simulink library "xpcdiamondlib"  (Simulink 6.0)
settings: Solver=ode45  SolverMode=SingleTasking  StartTime=0.0  StopTime=10.0  RelTol=1e-3
values from neighbouring files (symbols this model uses):
  channel = Channels(i)    [madadvpcl812.m]    (also in madadvpcl818.m; madhsad512.m; madsbsip16adc.m = round(channel); madsbsiphiadc.m = round(channel))
undefined symbols (not defined in the file or in its folder): maddiamondmm, maddiamondmm32, maddiamondmm32frame, maddsmm16at, madprometheus, mdadiamondmm, mdadiamondmmx, mdadsmm16at, mdaprometheus, mdidiamondmm, mdiodiamondquartz, mdiodsmm, mdodiamondmm, mdsrubymm, mdsrubymm1612, mdsrubymm416, misa8255
libraries: xpcmeasurementcomputinglib x12
(part 2 of 2)

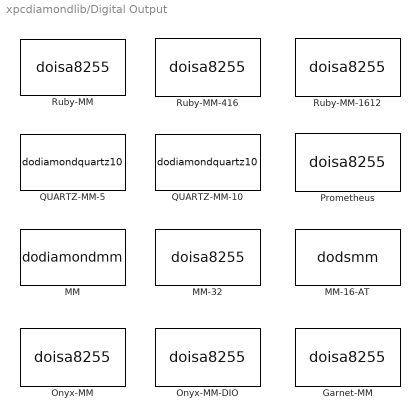
== system xpcdiamondlib/Digital Output ==
  "Garnet-MM " : S-Function  InitFcn=misa8255(1)  FunctionName=doisa8255  Parameters=channel, port, reset, initValue, sampletime, baseaddress, control  mask(dodsgarnetmm){channel=[1], port=A, reset=[1], initValue=[0], chip=1, sampletime=.001, baseaddress=0x300}
      mask prompts: channel "Channel vector:"; reset "Reset vector:"; initValue "Initial value vector:"; sampletime "Sample time:"; baseaddress "Base address (e.g. 0x300):"
      mask help:
      | Garnet-MM
      | Diamond Systems
      | Digital Output
      mask init:
      | baseaddress=hex2dec(baseaddress(3:end));
      | control=155;
      | [baseaddress,control,maskdisplay,maskdescription,reset,initValue]=misa8255(2, chip, port, channel, baseaddress, reset, initValue);
      | set_param(gcb, 'MaskDisplay', maskdisplay);
      | set_param(gcb, 'MaskDescription', maskdescription);
      mask Help: helpview(fullfile(docroot, 'mapfiles', 'xpc.map'), 'Diamond_Garnet-MM_DOUT')
      mask StyleString: edit,popup(A|B|C),edit,edit,popup(1|2),edit,edit
      mask Display: disp('Garnet-MM\nDiamond\nDigital Output');port_label('input',1,'1');
  "MM " : S-Function  InitFcn=mdodiamondmm(1);  FunctionName=dodiamondmm  Parameters=channel, reset, initValue, sampleTime, baseDec  mask(dodiamondmm){channel=[1], reset=[0 ], initValue=[1 ], sampleTime=0.001, base=0x300}
      mask prompts: channel "Channel vector:"; reset "Reset vector:"; initValue "Initial value vector:"; sampleTime "Sample time:"; base "Base address (e.g. 0x300):"
      mask help:
      | MM
      | Diamond
      | Digital Output
      mask init:
      | phase = 2;
      | [reset, initValue, baseDec, maskDisplay, maskDescription] = mdodiamondmm(phase, channel, reset, initValue, sampleTime, base);
      | set_param(gcb, 'MaskDisplay', maskDisplay);
      | set_param(gcb, 'MaskDescription', maskDescription);
      mask Help: helpview(fullfile(docroot, 'mapfiles', 'xpc.map'), 'Diamond_MM_DOUT')
      mask Display: disp('MM\nDiamond\nDigital Output'); port_label('input', 1, '1');
  "MM-16-AT " : S-Function  InitFcn=mdiodsmm(1, 'MM-16-AT', 'output');  FunctionName=dodsmm  Parameters=channel, reset, initValue, sampleTime, baseDec  mask(dodiamondmm16at){channel=[1], reset=[0 ], initValue=[1 ], sampleTime=0.001, baseHex=0x300}
      mask prompts: channel "Channel vector:"; reset "Reset vector:"; initValue "Initial value vector:"; sampleTime "Sample time:"; baseHex "Base address (e.g. 0x300):"
      mask help:
      | MM-16-AT
      | Diamond
      | Digital Output
      mask init:
      | phase = 2;
      | deviceName = 'MM-16-AT';
      | direction = 'output';
      | [baseDec, maskDisplay, maskDescription, reset, initValue] = mdiodsmm(phase, deviceName, direction, channel, sampleTime, baseHex, reset, initValue);
      | set_param(gcb, 'MaskDisplay', maskDisplay);
      | set_param(gcb, 'MaskDescription', maskDescription);
      mask Help: helpview(fullfile(docroot, 'mapfiles', 'xpc.map'), 'Diamond_MM-16-AT_DOUT')
      mask Display: disp('MM-16-AT\nDiamond\nDigital Output'); port_label('input', 1, '1');
  "MM-32 " : S-Function  InitFcn=misa8255(1)  FunctionName=doisa8255  Parameters=channel, port, reset, initValue, sampletime, baseaddress, control  mask(dodsmm32){channel=[1], port=A, reset=[1], initValue=[0], chip=1, sampletime=0.001, baseaddress=0x300}
      mask prompts: channel "Channel vector:"; reset "Reset vector:"; initValue "Initial value vector:"; sampletime "Sample time:"; baseaddress "Base address (i.e. 0xd000):"
      mask help:
      | MM-32
      | Diamond Systems
      | Digital Output
      mask init:
      | baseaddress=hex2dec(baseaddress(3:end));
      | control=155;
      | boardType=16;
      | [baseaddress,control,maskdisplay,maskdescription,reset,initValue]=misa8255(2, chip, port, channel, baseaddress, reset, initValue);
      | set_param(gcb, 'MaskDisplay', maskdisplay);
      | set_param(gcb, 'MaskDescription', maskdescription);
      mask Help: helpview(fullfile(docroot, 'mapfiles', 'xpc.map'), 'Diamond_MM-32_DOUT')
      mask StyleString: edit,popup(A|B|C),edit,edit,popup(1),edit,edit
      mask Display: disp('MM-32\nDiamond\nDigital Output');port_label('input',1,'1');
  "Onyx-MM " : S-Function  InitFcn=misa8255(1)  FunctionName=doisa8255  Parameters=channel, port, reset, initValue, sampletime, baseaddress, control  mask(dodsonyxmm){channel=[1], port=A, reset=[1], initValue=[0], chip=1, sampletime=.001, baseaddress=0x300}
      mask prompts: channel "Channel vector:"; reset "Reset vector:"; initValue "Initial value vector:"; sampletime "Sample time:"; baseaddress "Base address (e.g. 0x300):"
      mask help:
      | Onyx-MM
      | Diamond Systems
      | Digital Output
      mask init: same as xpcdiamondlib/Digital Output/MM-32 
      mask Help: helpview(fullfile(docroot, 'mapfiles', 'xpc.map'), 'Diamond_Onyx-MM_DOUT')
      mask StyleString: edit,popup(A|B|C),edit,edit,popup(1|2),edit,edit
      mask Display: disp('Onyx-MM\nDiamond\nDigital Output');port_label('input',1,'1');
  "Onyx-MM-DIO " : S-Function  InitFcn=misa8255(1)  FunctionName=doisa8255  Parameters=channel, port, reset, initValue, sampletime, baseaddress, control  mask(dodsonyxmmdio){channel=[1], port=A, reset=[1], initValue=[0], chip=1, sampletime=.001, baseaddress=0x300}
      mask prompts: channel "Channel vector:"; reset "Reset vector:"; initValue "Initial value vector:"; sampletime "Sample time:"; baseaddress "Base address (e.g. 0x300):"
      mask help:
      | Onyx-MM-DIO
      | Diamond Systems
      | Digital Output
      mask init: same as xpcdiamondlib/Digital Output/Garnet-MM 
      mask Help: helpview(fullfile(docroot, 'mapfiles', 'xpc.map'), 'Diamond_Onyx-MM-DIO_DOUT')
      mask StyleString: edit,popup(A|B|C),edit,edit,popup(1|2),edit,edit
      mask Display: disp('Onyx-MM-DIO\nDiamond\nDigital Output');port_label('input',1,'1');
  Prometheus : S-Function  InitFcn=misa8255(1)  FunctionName=doisa8255  Parameters=channel, port, reset, initValue, sampletime, baseaddress, control  mask(dodsprometheus){channel=[1], port=B, reset=[1], initValue=[0 ], chip=1, sampletime=0.001, baseaddress=0x280}
      mask prompts: channel "Channel vector:"; reset "Reset vector:"; initValue "Initial value vector:"; sampletime "Sample time:"; baseaddress "Base address (e.g. 0x280):"
      mask help:
      | Prometheus
      | Diamond Systems
      | Digital Output
      mask init: same as xpcdiamondlib/Digital Output/MM-32 
      mask Help: helpview(fullfile(docroot, 'mapfiles', 'xpc.map'), 'Diamond_Prometheus_DOUT')
      mask StyleString: edit,popup(A|B|C),edit,edit,popup(1),edit,edit
      mask Display: disp('Prometheus\nDiamond\nDigital Output');port_label('input',1,'1');
  "QUARTZ-MM-10 " : S-Function  InitFcn=mdiodiamondquartz(1);  FunctionName=dodiamondquartz10  Parameters=channel, ts, baseAddress  mask(dodiamondquartz10){channel=[1], ts=0.001, baseAddressIn=0x300}
      mask prompts: channel "Channel vector:"; ts "Sample time:"; baseAddressIn "Base address (i.e. 0xd000):"
      mask help:
      | QUARTZ-MM-10
      | Diamond Systems
      | Digital Output
      mask init:
      | type=1;
      | baseAddress=768;
      | [baseAddress, maskdisplay,maskdescription]=mdiodiamondquartz(2, type, channel, baseAddressIn);
      | set_param(gcb,'MaskDisplay',maskdisplay);
      | set_param(gcb,'MaskDescription',maskdescription);
      mask Help: helpview(fullfile(docroot, 'mapfiles', 'xpc.map'), 'Diamond_QUARTZ-MM-10_DOUT')
      mask Display: disp('Quartz-MM-10\nDiamond\nDigital Output'); port_label('input', 1, '1');
  "QUARTZ-MM-5 " : S-Function  InitFcn=mdiodiamondquartz(1);  FunctionName=dodiamondquartz10  Parameters=channel, ts, baseAddress  mask(dodiamondquartz10){channel=[1], ts=0.001, baseAddressIn=0x300}
      mask prompts: channel "Channel vector:"; ts "Sample time:"; baseAddressIn "Base address (i.e. 0xd000):"
      mask help:
      | Quartz-MM-5
      | Diamond
      | Digital Output
      mask init:
      | type=3;
      | baseAddress=768;
      | [baseAddress, maskdisplay,maskdescription]=mdiodiamondquartz(2, type, channel, baseAddressIn);
      | set_param(gcb,'MaskDisplay',maskdisplay);
      | set_param(gcb,'MaskDescription',maskdescription);
      mask Help: helpview(fullfile(docroot, 'mapfiles', 'xpc.map'), 'Diamond_QUARTZ-MM-5_DOUT')
      mask Display: disp('Quartz-MM-5\nDiamond\nDigital Output'); port_label('input', 1, '1');
  "Ruby-MM " : S-Function  InitFcn=misa8255(1)  FunctionName=doisa8255  Parameters=channel, port, reset, initValue, sampletime, baseaddress, control  mask(dodsrubymm){channel=[1], port=A, reset=[1], initValue=[0], chip=1, sampletime=0.001, baseaddress=0x300}
      mask prompts: channel "Channel vector:"; reset "Reset vector:"; initValue "Initial value vector:"; sampletime "Sample time:"; baseaddress "Base address (i.e. 0xd000):"
      mask help:
      | Ruby-MM
      | Diamond Systems
      | Digital Output
      mask init: same as xpcdiamondlib/Digital Output/Garnet-MM 
      mask Help: helpview(fullfile(docroot, 'mapfiles', 'xpc.map'), 'Diamond_Ruby-MM_DOUT')
      mask StyleString: edit,popup(A|B|C),edit,edit,popup(1),edit,edit
      mask Display: disp('Ruby-MM\nDiamond\nDigital Output');port_label('input',1,'1');
  "Ruby-MM-1612 " : S-Function  InitFcn=misa8255(1)  FunctionName=doisa8255  Parameters=channel, port, reset, initValue, sampletime, baseaddress, control  mask(dodsrubymm1612){channel=[1], port=A, reset=[1], initValue=[0], chip=1, sampletime=.001, baseaddress=0x300}
      mask prompts: channel "Channel vector:"; reset "Reset vector:"; initValue "Initial value vector:"; sampletime "Sample time:"; baseaddress "Base address (e.g. 0x300):"
      mask help:
      | Ruby-MM-1612
      | Diamond Systems
      | Digital Output
      mask init: same as xpcdiamondlib/Digital Output/MM-32 
      mask Help: helpview(fullfile(docroot, 'mapfiles', 'xpc.map'), 'Diamond_Ruby-MM-1612_DOUT')
      mask StyleString: edit,popup(A|B|C),edit,edit,popup(1),edit,edit
      mask Display: disp('Ruby-MM-1612\nDiamond\nDigital Output');port_label('input',1,'1');
  "Ruby-MM-416 " : S-Function  InitFcn=misa8255(1)  FunctionName=doisa8255  Parameters=channel, port, reset, initValue, sampletime, baseaddress, control  mask(dodsrubymm416){channel=[1], port=A, reset=[1], initValue=[0], chip=1, sampletime=.001, baseaddress=0x300}
      mask prompts: channel "Channel vector:"; reset "Reset vector:"; initValue "Initial value vector:"; sampletime "Sample time:"; baseaddress "Base address (e.g. 0x300):"
      mask help:
      | Ruby-MM-416
      | Diamond Systems
      | Digital Output
      mask init: same as xpcdiamondlib/Digital Output/MM-32 
      mask Help: helpview(fullfile(docroot, 'mapfiles', 'xpc.map'), 'Diamond_Ruby-MM-416_DOUT')
      mask StyleString: edit,popup(A|B|C),edit,edit,popup(1),edit,edit
      mask Display: disp('Ruby-MM-416\nDiamond\nDigital Output');port_label('input',1,'1');

== system xpcdiamondlib/RS232 ==

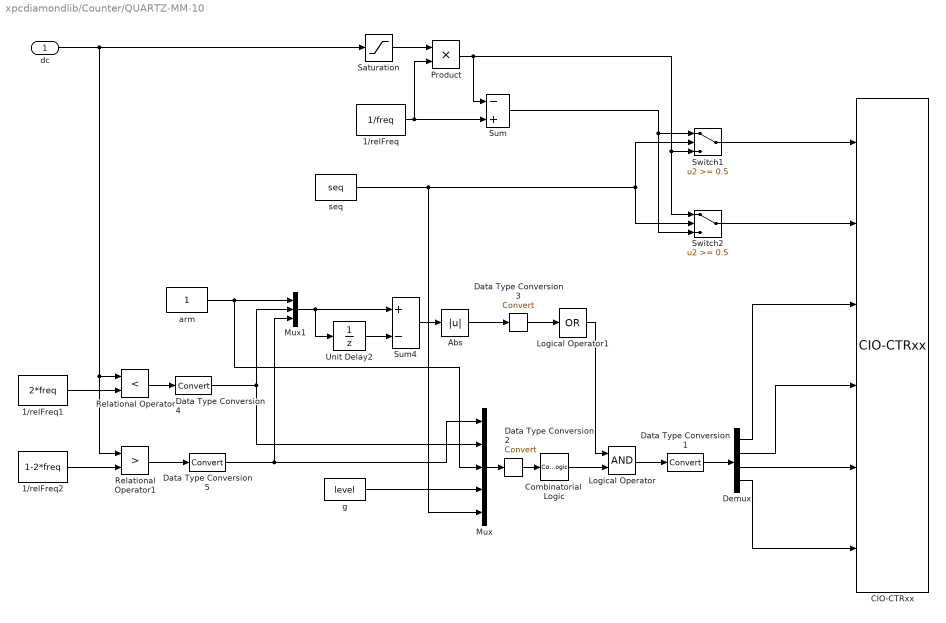
== system xpcdiamondlib/Counter/QUARTZ-MM-10  ==
  dc : Inport  LatchInput=off
  1/relFreq : Constant  Value=1/freq
  1/relFreq1 : Constant  Value=2*freq
  1/relFreq2 : Constant  Value=1-2*freq
  Abs : Abs  SaturateOnIntegerOverflow=on
  "CIO-CTRxx " : xpcmeasurementcomputinglib/Counter/CIO-CTRxx   mastermode=MasterMode  countermode=CounterMode  init=Init  commands=Runtime  term=Term  ts=Ts  baseAddress=baseAddress
  Combinatorial  Logic : CombinatorialLogic  TruthTable=[0,0,1,0;0,0,1,0;0,0,0,1;0,0,0,1;0,1,0,0;1,0,0,0;0,1,0,0;1,0,0,0;0,0,1,0;0,0,1,0;0,0,0,1;0,0,0,1;0,0,1,0;0,0,1,0;0,0,1,0;0,0,1,0;0,0,1,0;0,0,1,0;0,0,0,1;0,0,0,1;0,0,0,1;0,0,0,1;0,0,0,1;0,0,0,1;0,0,0,0;0,0,0,0;0,0,0,0;0,0,0,0;0,0,0,0;0,0,0,0;0,0,0,0;0,0,0,0]
  Data Type Conversion1 : DataTypeConversion  SaturateOnIntegerOverflow=on  RndMeth=Zero
  Data Type Conversion2 : DataTypeConversion  SaturateOnIntegerOverflow=on  RndMeth=Zero
  Data Type Conversion3 : DataTypeConversion  SaturateOnIntegerOverflow=on  RndMeth=Zero
  Data Type Conversion4 : DataTypeConversion  OutDataTypeMode=double  SaturateOnIntegerOverflow=on  RndMeth=Zero
  Data Type Conversion5 : DataTypeConversion  OutDataTypeMode=double  SaturateOnIntegerOverflow=on  RndMeth=Zero
  Demux : Demux
  Logical Operator : Logic
  Logical Operator1 : Logic  Operator=OR  Inputs=1
  Mux : Mux  Inputs=5
  Mux1 : Mux  Inputs=3
  Product : Product  SaturateOnIntegerOverflow=on  InputSameDT=on
  Relational Operator : RelationalOperator  Operator=<  InputSameDT=on
  Relational Operator1 : RelationalOperator  Operator=>  InputSameDT=on
  Saturation : Saturate  UpperLimit=1-2*freq  LowerLimit=2*freq  ZeroCross=off
  Sum : Sum  Inputs=-+  SaturateOnIntegerOverflow=on  InputSameDT=on
  Sum4 : Sum  Inputs=+-  SaturateOnIntegerOverflow=on  InputSameDT=on
  Switch1 : Switch  Threshold=0.5  InputSameDT=on
  Switch2 : Switch  Threshold=0.5  InputSameDT=on
  Unit Delay2 : UnitDelay  X0=2  SampleTime=Ts
  arm : Constant
  g : Constant  Value=level
  seq : Constant  Value=seq
  wires:
  Data Type Conversion5/1 -> Mux1/3, Mux/1
  Data Type Conversion4/1 -> Mux1/2, Mux/2
  Data Type Conversion3/1 -> Logical Operator1/1
  Data Type Conversion2/1 -> Combinatorial  Logic/1
  Data Type Conversion1/1 -> Demux/1
  1/relFreq1/1 -> Relational Operator/2
  1/relFreq/1 -> Product/2, Sum/2
  Product/1 -> Sum/1, Switch1/3, Switch2/1
  1/relFreq2/1 -> Relational Operator1/2
  Relational Operator1/1 -> Data Type Conversion5/1
  Relational Operator/1 -> Data Type Conversion4/1
  Combinatorial  Logic/1 -> Logical Operator/2
  Logical Operator/1 -> Data Type Conversion1/1
  Unit Delay2/1 -> Sum4/2
  Sum4/1 -> Abs/1
  Logical Operator1/1 -> Logical Operator/1
  Demux/1 -> "CIO-CTRxx "/3
  Demux/2 -> "CIO-CTRxx "/4
  Demux/3 -> "CIO-CTRxx "/5
  Demux/4 -> "CIO-CTRxx "/6
  g/1 -> Mux/4
  seq/1 -> Switch1/2, Switch2/2, Mux/5
  Sum/1 -> Switch1/1, Switch2/3
  Saturation/1 -> Product/1
  dc/1 -> Saturation/1, Relational Operator/1, Relational Operator1/1
  Mux1/1 -> Sum4/1, Unit Delay2/1
  arm/1 -> Mux1/1, Mux/3
  Abs/1 -> Data Type Conversion3/1
  Mux/1 -> Data Type Conversion2/1
  Switch1/1 -> "CIO-CTRxx "/1
  Switch2/1 -> "CIO-CTRxx "/2

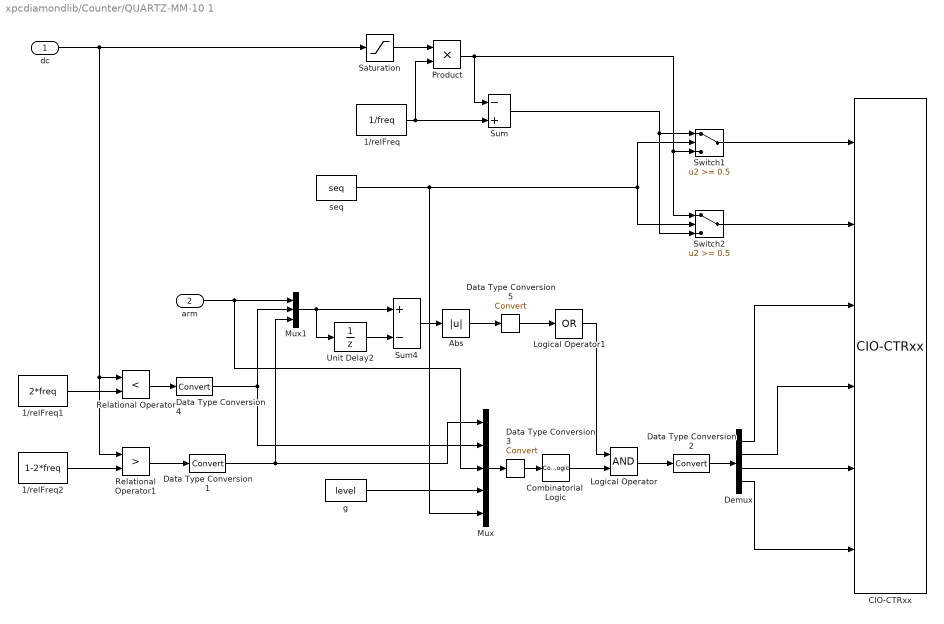
== system xpcdiamondlib/Counter/QUARTZ-MM-10 1 ==
  dc : Inport  LatchInput=off
  arm : Inport  Port=2  LatchInput=off
  1/relFreq : Constant  Value=1/freq
  1/relFreq1 : Constant  Value=2*freq
  1/relFreq2 : Constant  Value=1-2*freq
  Abs : Abs  SaturateOnIntegerOverflow=on
  "CIO-CTRxx " : xpcmeasurementcomputinglib/Counter/CIO-CTRxx   mastermode=MasterMode  countermode=CounterMode  init=Init  commands=Runtime  term=Term  ts=Ts  baseAddress=baseAddress
  Combinatorial  Logic : CombinatorialLogic  TruthTable=[0,0,1,0;0,0,1,0;0,0,0,1;0,0,0,1;0,1,0,0;1,0,0,0;0,1,0,0;1,0,0,0;0,0,1,0;0,0,1,0;0,0,0,1;0,0,0,1;0,0,1,0;0,0,1,0;0,0,1,0;0,0,1,0;0,0,1,0;0,0,1,0;0,0,0,1;0,0,0,1;0,0,0,1;0,0,0,1;0,0,0,1;0,0,0,1;0,0,0,0;0,0,0,0;0,0,0,0;0,0,0,0;0,0,0,0;0,0,0,0;0,0,0,0;0,0,0,0]
  Data Type Conversion1 : DataTypeConversion  OutDataTypeMode=double  SaturateOnIntegerOverflow=on  RndMeth=Zero
  Data Type Conversion2 : DataTypeConversion  SaturateOnIntegerOverflow=on  RndMeth=Zero
  Data Type Conversion3 : DataTypeConversion  SaturateOnIntegerOverflow=on  RndMeth=Zero
  Data Type Conversion4 : DataTypeConversion  OutDataTypeMode=double  SaturateOnIntegerOverflow=on  RndMeth=Zero
  Data Type Conversion5 : DataTypeConversion  SaturateOnIntegerOverflow=on  RndMeth=Zero
  Demux : Demux
  Logical Operator : Logic
  Logical Operator1 : Logic  Operator=OR  Inputs=1
  Mux : Mux  Inputs=5
  Mux1 : Mux  Inputs=3
  Product : Product  SaturateOnIntegerOverflow=on  InputSameDT=on
  Relational Operator : RelationalOperator  Operator=<  InputSameDT=on
  Relational Operator1 : RelationalOperator  Operator=>  InputSameDT=on
  Saturation : Saturate  UpperLimit=1-2*freq  LowerLimit=2*freq  ZeroCross=off
  Sum : Sum  Inputs=-+  SaturateOnIntegerOverflow=on  InputSameDT=on
  Sum4 : Sum  Inputs=+-  SaturateOnIntegerOverflow=on  InputSameDT=on
  Switch1 : Switch  Threshold=0.5  InputSameDT=on
  Switch2 : Switch  Threshold=0.5  InputSameDT=on
  Unit Delay2 : UnitDelay  X0=2  SampleTime=Ts
  g : Constant  Value=level
  seq : Constant  Value=seq
  wires:
  Data Type Conversion5/1 -> Logical Operator1/1
  Data Type Conversion3/1 -> Combinatorial  Logic/1
  Data Type Conversion2/1 -> Demux/1
  Data Type Conversion1/1 -> Mux1/3, Mux/1
  Data Type Conversion4/1 -> Mux1/2, Mux/2
  1/relFreq1/1 -> Relational Operator/2
  1/relFreq/1 -> Product/2, Sum/2
  Product/1 -> Sum/1, Switch1/3, Switch2/1
  1/relFreq2/1 -> Relational Operator1/2
  Relational Operator1/1 -> Data Type Conversion1/1
  Relational Operator/1 -> Data Type Conversion4/1
  Combinatorial  Logic/1 -> Logical Operator/2
  Logical Operator/1 -> Data Type Conversion2/1
  Unit Delay2/1 -> Sum4/2
  Sum4/1 -> Abs/1
  Logical Operator1/1 -> Logical Operator/1
  Demux/1 -> "CIO-CTRxx "/3
  Demux/2 -> "CIO-CTRxx "/4
  Demux/3 -> "CIO-CTRxx "/5
  Demux/4 -> "CIO-CTRxx "/6
  g/1 -> Mux/4
  seq/1 -> Switch1/2, Switch2/2, Mux/5
  Sum/1 -> Switch1/1, Switch2/3
  Saturation/1 -> Product/1
  dc/1 -> Saturation/1, Relational Operator/1, Relational Operator1/1
  Mux1/1 -> Sum4/1, Unit Delay2/1
  arm/1 -> Mux1/1, Mux/3
  Abs/1 -> Data Type Conversion5/1
  Mux/1 -> Data Type Conversion3/1
  Switch1/1 -> "CIO-CTRxx "/1
  Switch2/1 -> "CIO-CTRxx "/2

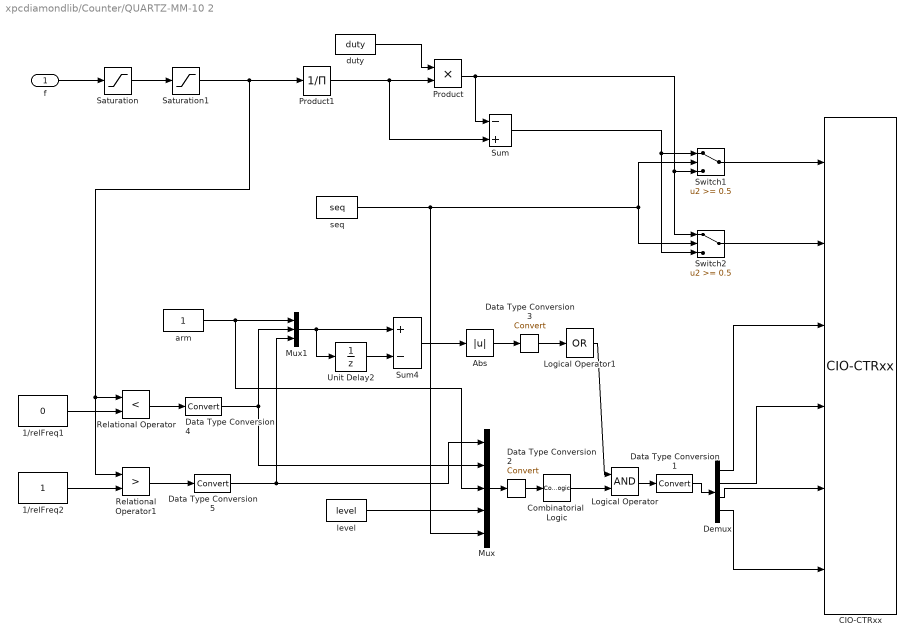
== system xpcdiamondlib/Counter/QUARTZ-MM-10 2 ==
  f : Inport  LatchInput=off
  1/relFreq1 : Constant  Value=0
  1/relFreq2 : Constant
  Abs : Abs  SaturateOnIntegerOverflow=on
  "CIO-CTRxx " : xpcmeasurementcomputinglib/Counter/CIO-CTRxx   mastermode=MasterMode  countermode=CounterMode  init=Init  commands=Runtime  term=Term  ts=Ts  baseAddress=baseAddress
  Combinatorial  Logic : CombinatorialLogic  TruthTable=[0,0,1,0;0,0,1,0;0,0,0,1;0,0,0,1;0,1,0,0;1,0,0,0;0,1,0,0;1,0,0,0;0,0,1,0;0,0,1,0;0,0,0,1;0,0,0,1;0,0,1,0;0,0,1,0;0,0,1,0;0,0,1,0;0,0,1,0;0,0,1,0;0,0,0,1;0,0,0,1;0,0,0,1;0,0,0,1;0,0,0,1;0,0,0,1;0,0,0,0;0,0,0,0;0,0,0,0;0,0,0,0;0,0,0,0;0,0,0,0;0,0,0,0;0,0,0,0]
  Data Type Conversion1 : DataTypeConversion  SaturateOnIntegerOverflow=on  RndMeth=Zero
  Data Type Conversion2 : DataTypeConversion  SaturateOnIntegerOverflow=on  RndMeth=Zero
  Data Type Conversion3 : DataTypeConversion  SaturateOnIntegerOverflow=on  RndMeth=Zero
  Data Type Conversion4 : DataTypeConversion  OutDataTypeMode=double  SaturateOnIntegerOverflow=on  RndMeth=Zero
  Data Type Conversion5 : DataTypeConversion  OutDataTypeMode=double  SaturateOnIntegerOverflow=on  RndMeth=Zero
  Demux : Demux
  Logical Operator : Logic
  Logical Operator1 : Logic  Operator=OR  Inputs=1
  Mux : Mux  Inputs=5
  Mux1 : Mux  Inputs=3
  Product : Product  SaturateOnIntegerOverflow=on  InputSameDT=on
  Product1 : Product  Inputs=/  SaturateOnIntegerOverflow=on  InputSameDT=on
  Relational Operator : RelationalOperator  Operator=<  InputSameDT=on
  Relational Operator1 : RelationalOperator  Operator=>  InputSameDT=on
  Saturation : Saturate  UpperLimit=duty/2  LowerLimit=duty/(2^16-1)  ZeroCross=off
  Saturation1 : Saturate  UpperLimit=(1-duty)/2  LowerLimit=(1-duty)/(2^16-1)  ZeroCross=off
  Sum : Sum  Inputs=-+  SaturateOnIntegerOverflow=on  InputSameDT=on
  Sum4 : Sum  Inputs=+-  SaturateOnIntegerOverflow=on  InputSameDT=on
  Switch1 : Switch  Threshold=0.5  InputSameDT=on
  Switch2 : Switch  Threshold=0.5  InputSameDT=on
  Unit Delay2 : UnitDelay  X0=2  SampleTime=Ts
  arm : Constant
  duty : Constant  Value=duty
  level : Constant  Value=level
  seq : Constant  Value=seq
  wires:
  Data Type Conversion5/1 -> Mux1/3, Mux/1
  Data Type Conversion4/1 -> Mux1/2, Mux/2
  Data Type Conversion3/1 -> Logical Operator1/1
  Data Type Conversion2/1 -> Combinatorial  Logic/1
  Data Type Conversion1/1 -> Demux/1
  1/relFreq1/1 -> Relational Operator/2
  Product/1 -> Sum/1, Switch1/3, Switch2/1
  1/relFreq2/1 -> Relational Operator1/2
  Relational Operator1/1 -> Data Type Conversion5/1
  Relational Operator/1 -> Data Type Conversion4/1
  Combinatorial  Logic/1 -> Logical Operator/2
  Logical Operator/1 -> Data Type Conversion1/1
  Unit Delay2/1 -> Sum4/2
  Sum4/1 -> Abs/1
  Logical Operator1/1 -> Logical Operator/1
  Demux/1 -> "CIO-CTRxx "/3
  Demux/2 -> "CIO-CTRxx "/4
  Demux/3 -> "CIO-CTRxx "/5
  Demux/4 -> "CIO-CTRxx "/6
  level/1 -> Mux/4
  Switch1/1 -> "CIO-CTRxx "/1
  Switch2/1 -> "CIO-CTRxx "/2
  seq/1 -> Switch1/2, Switch2/2, Mux/5
  Sum/1 -> Switch1/1, Switch2/3
  Saturation/1 -> Saturation1/1
  f/1 -> Saturation/1
  Mux1/1 -> Sum4/1, Unit Delay2/1
  arm/1 -> Mux1/1, Mux/3
  Abs/1 -> Data Type Conversion3/1
  Mux/1 -> Data Type Conversion2/1
  Saturation1/1 -> Product1/1, Relational Operator1/1, Relational Operator/1
  duty/1 -> Product/1
  Product1/1 -> Product/2, Sum/2

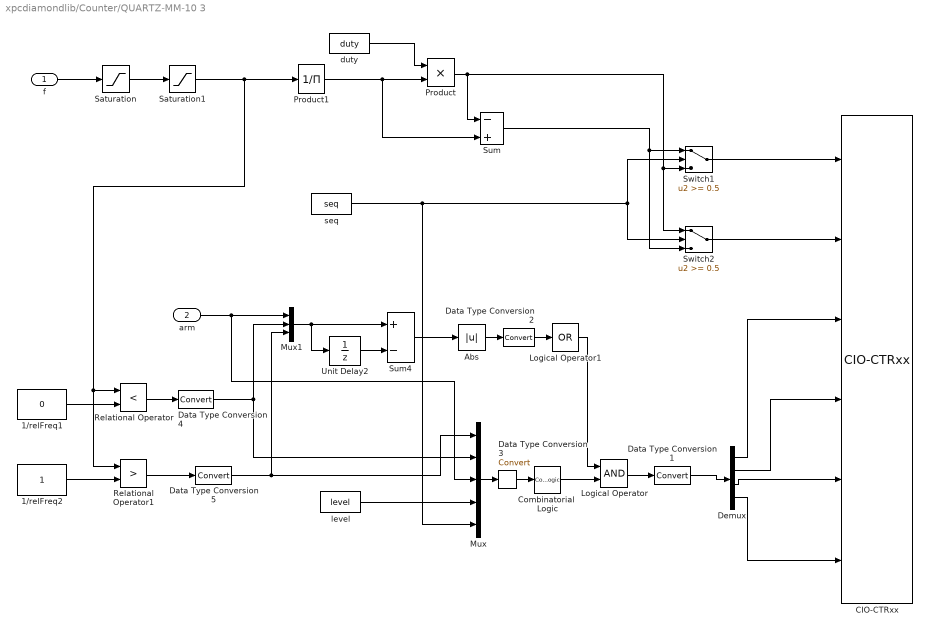
== system xpcdiamondlib/Counter/QUARTZ-MM-10 3 ==
  f : Inport  LatchInput=off
  arm : Inport  Port=2  LatchInput=off
  1/relFreq1 : Constant  Value=0
  1/relFreq2 : Constant
  Abs : Abs  SaturateOnIntegerOverflow=on
  "CIO-CTRxx " : xpcmeasurementcomputinglib/Counter/CIO-CTRxx   mastermode=MasterMode  countermode=CounterMode  init=Init  commands=Runtime  term=Term  ts=Ts  baseAddress=baseAddress
  Combinatorial  Logic : CombinatorialLogic  TruthTable=[0,0,1,0;0,0,1,0;0,0,0,1;0,0,0,1;0,1,0,0;1,0,0,0;0,1,0,0;1,0,0,0;0,0,1,0;0,0,1,0;0,0,0,1;0,0,0,1;0,0,1,0;0,0,1,0;0,0,1,0;0,0,1,0;0,0,1,0;0,0,1,0;0,0,0,1;0,0,0,1;0,0,0,1;0,0,0,1;0,0,0,1;0,0,0,1;0,0,0,0;0,0,0,0;0,0,0,0;0,0,0,0;0,0,0,0;0,0,0,0;0,0,0,0;0,0,0,0]
  Data Type Conversion1 : DataTypeConversion  SaturateOnIntegerOverflow=on  RndMeth=Zero
  Data Type Conversion2 : DataTypeConversion  SaturateOnIntegerOverflow=on  RndMeth=Zero
  Data Type Conversion3 : DataTypeConversion  SaturateOnIntegerOverflow=on  RndMeth=Zero
  Data Type Conversion4 : DataTypeConversion  OutDataTypeMode=double  SaturateOnIntegerOverflow=on  RndMeth=Zero
  Data Type Conversion5 : DataTypeConversion  OutDataTypeMode=double  SaturateOnIntegerOverflow=on  RndMeth=Zero
  Demux : Demux
  Logical Operator : Logic
  Logical Operator1 : Logic  Operator=OR  Inputs=1
  Mux : Mux  Inputs=5
  Mux1 : Mux  Inputs=3
  Product : Product  SaturateOnIntegerOverflow=on  InputSameDT=on
  Product1 : Product  Inputs=/  SaturateOnIntegerOverflow=on  InputSameDT=on
  Relational Operator : RelationalOperator  Operator=<  InputSameDT=on
  Relational Operator1 : RelationalOperator  Operator=>  InputSameDT=on
  Saturation : Saturate  UpperLimit=duty/2  LowerLimit=duty/(2^16-1)  ZeroCross=off
  Saturation1 : Saturate  UpperLimit=(1-duty)/2  LowerLimit=(1-duty)/(2^16-1)  ZeroCross=off
  Sum : Sum  Inputs=-+  SaturateOnIntegerOverflow=on  InputSameDT=on
  Sum4 : Sum  Inputs=+-  SaturateOnIntegerOverflow=on  InputSameDT=on
  Switch1 : Switch  Threshold=0.5  InputSameDT=on
  Switch2 : Switch  Threshold=0.5  InputSameDT=on
  Unit Delay2 : UnitDelay  X0=2  SampleTime=Ts
  duty : Constant  Value=duty
  level : Constant  Value=level
  seq : Constant  Value=seq
  wires:
  Data Type Conversion5/1 -> Mux1/3, Mux/1
  Data Type Conversion4/1 -> Mux1/2, Mux/2
  Data Type Conversion3/1 -> Combinatorial  Logic/1
  Data Type Conversion2/1 -> Logical Operator1/1
  Data Type Conversion1/1 -> Demux/1
  1/relFreq1/1 -> Relational Operator/2
  Product/1 -> Sum/1, Switch1/3, Switch2/1
  1/relFreq2/1 -> Relational Operator1/2
  Relational Operator1/1 -> Data Type Conversion5/1
  Relational Operator/1 -> Data Type Conversion4/1
  Combinatorial  Logic/1 -> Logical Operator/2
  Logical Operator/1 -> Data Type Conversion1/1
  Unit Delay2/1 -> Sum4/2
  Sum4/1 -> Abs/1
  Logical Operator1/1 -> Logical Operator/1
  Demux/1 -> "CIO-CTRxx "/3
  Demux/2 -> "CIO-CTRxx "/4
  Demux/3 -> "CIO-CTRxx "/5
  Demux/4 -> "CIO-CTRxx "/6
  level/1 -> Mux/4
  Switch1/1 -> "CIO-CTRxx "/1
  Switch2/1 -> "CIO-CTRxx "/2
  seq/1 -> Switch1/2, Switch2/2, Mux/5
  Sum/1 -> Switch1/1, Switch2/3
  Saturation/1 -> Saturation1/1
  f/1 -> Saturation/1
  Mux1/1 -> Sum4/1, Unit Delay2/1
  arm/1 -> Mux1/1, Mux/3
  Abs/1 -> Data Type Conversion2/1
  Mux/1 -> Data Type Conversion3/1
  Saturation1/1 -> Product1/1, Relational Operator1/1, Relational Operator/1
  duty/1 -> Product/1
  Product1/1 -> Product/2, Sum/2

== system xpcdiamondlib/Counter/QUARTZ-MM-10 4 ==
  "CIO-CTRxx " : xpcmeasurementcomputinglib/Counter/CIO-CTRxx   mastermode=MasterMode  countermode=CounterMode  init=Init  commands=Runtime  term=Term  ts=Ts  baseAddress=baseAddress
  Demux : Demux  Outputs=2
  Product : Product  Inputs=/  SaturateOnIntegerOverflow=on  InputSameDT=on
  Product1 : Product  Inputs=**  SaturateOnIntegerOverflow=on  InputSameDT=on
  f : Outport
  dc : Outport  Port=2
  wires:
  "CIO-CTRxx "/1 -> Demux/1
  Product1/1 -> dc/1
  Product/1 -> Product1/2, f/1
  Demux/2 -> Product/1
  Demux/1 -> Product1/1

== system xpcdiamondlib/Counter/QUARTZ-MM-10 5 ==
  "CIO-CTRxx " : xpcmeasurementcomputinglib/Counter/CIO-CTRxx   mastermode=MasterMode  countermode=CounterMode  init=Init  commands=Runtime  term=Term  ts=Ts  baseAddress=baseAddress
  Product : Product  Inputs=/  SaturateOnIntegerOverflow=on  InputSameDT=on
  f : Outport
  wires:
  Product/1 -> f/1
  "CIO-CTRxx "/1 -> Product/1

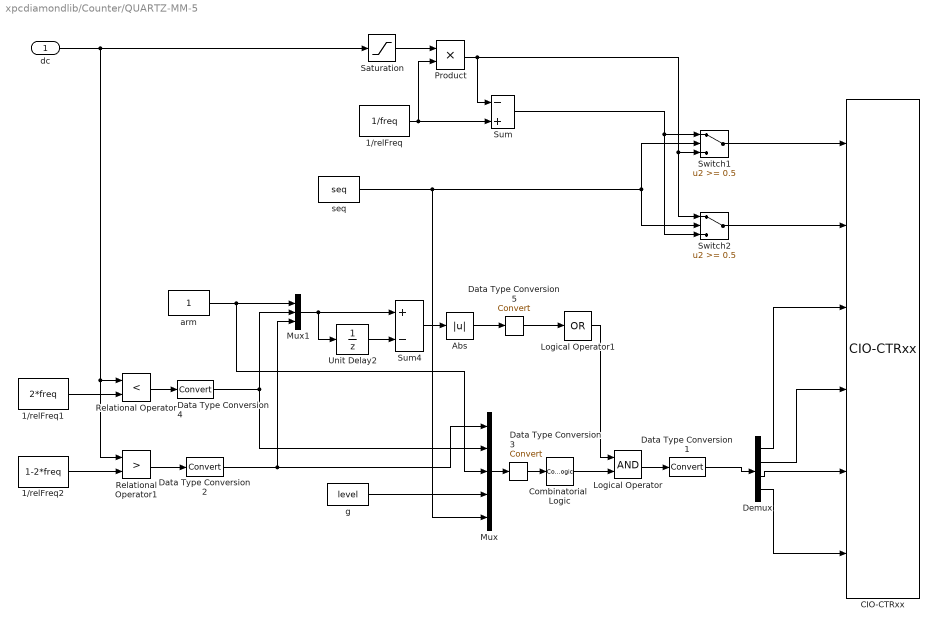
== system xpcdiamondlib/Counter/QUARTZ-MM-5  ==
  dc : Inport  LatchInput=off
  1/relFreq : Constant  Value=1/freq
  1/relFreq1 : Constant  Value=2*freq
  1/relFreq2 : Constant  Value=1-2*freq
  Abs : Abs  SaturateOnIntegerOverflow=on
  "CIO-CTRxx " : xpcmeasurementcomputinglib/Counter/CIO-CTRxx   mastermode=MasterMode  countermode=CounterMode  init=Init  commands=Runtime  term=Term  ts=Ts  baseAddress=baseAddress
  Combinatorial  Logic : CombinatorialLogic  TruthTable=[0,0,1,0;0,0,1,0;0,0,0,1;0,0,0,1;0,1,0,0;1,0,0,0;0,1,0,0;1,0,0,0;0,0,1,0;0,0,1,0;0,0,0,1;0,0,0,1;0,0,1,0;0,0,1,0;0,0,1,0;0,0,1,0;0,0,1,0;0,0,1,0;0,0,0,1;0,0,0,1;0,0,0,1;0,0,0,1;0,0,0,1;0,0,0,1;0,0,0,0;0,0,0,0;0,0,0,0;0,0,0,0;0,0,0,0;0,0,0,0;0,0,0,0;0,0,0,0]
  Data Type Conversion1 : DataTypeConversion  SaturateOnIntegerOverflow=on  RndMeth=Zero
  Data Type Conversion2 : DataTypeConversion  OutDataTypeMode=double  SaturateOnIntegerOverflow=on  RndMeth=Zero
  Data Type Conversion3 : DataTypeConversion  SaturateOnIntegerOverflow=on  RndMeth=Zero
  Data Type Conversion4 : DataTypeConversion  OutDataTypeMode=double  SaturateOnIntegerOverflow=on  RndMeth=Zero
  Data Type Conversion5 : DataTypeConversion  SaturateOnIntegerOverflow=on  RndMeth=Zero
  Demux : Demux
  Logical Operator : Logic
  Logical Operator1 : Logic  Operator=OR  Inputs=1
  Mux : Mux  Inputs=5
  Mux1 : Mux  Inputs=3
  Product : Product  SaturateOnIntegerOverflow=on  InputSameDT=on
  Relational Operator : RelationalOperator  Operator=<  InputSameDT=on
  Relational Operator1 : RelationalOperator  Operator=>  InputSameDT=on
  Saturation : Saturate  UpperLimit=1-2*freq  LowerLimit=2*freq  ZeroCross=off
  Sum : Sum  Inputs=-+  SaturateOnIntegerOverflow=on  InputSameDT=on
  Sum4 : Sum  Inputs=+-  SaturateOnIntegerOverflow=on  InputSameDT=on
  Switch1 : Switch  Threshold=0.5  InputSameDT=on
  Switch2 : Switch  Threshold=0.5  InputSameDT=on
  Unit Delay2 : UnitDelay  X0=2  SampleTime=Ts
  arm : Constant
  g : Constant  Value=level
  seq : Constant  Value=seq
  wires:
  Data Type Conversion5/1 -> Logical Operator1/1
  Data Type Conversion3/1 -> Combinatorial  Logic/1
  Data Type Conversion1/1 -> Demux/1
  Data Type Conversion2/1 -> Mux/1, Mux1/3
  Data Type Conversion4/1 -> Mux/2, Mux1/2
  Switch2/1 -> "CIO-CTRxx "/2
  Switch1/1 -> "CIO-CTRxx "/1
  Mux/1 -> Data Type Conversion3/1
  Abs/1 -> Data Type Conversion5/1
  arm/1 -> Mux/3, Mux1/1
  Mux1/1 -> Unit Delay2/1, Sum4/1
  dc/1 -> Relational Operator1/1, Relational Operator/1, Saturation/1
  Saturation/1 -> Product/1
  Sum/1 -> Switch2/3, Switch1/1
  seq/1 -> Mux/5, Switch2/2, Switch1/2
  g/1 -> Mux/4
  Demux/4 -> "CIO-CTRxx "/6
  Demux/3 -> "CIO-CTRxx "/5
  Demux/2 -> "CIO-CTRxx "/4
  Demux/1 -> "CIO-CTRxx "/3
  Logical Operator1/1 -> Logical Operator/1
  Sum4/1 -> Abs/1
  Unit Delay2/1 -> Sum4/2
  Logical Operator/1 -> Data Type Conversion1/1
  Combinatorial  Logic/1 -> Logical Operator/2
  Relational Operator/1 -> Data Type Conversion4/1
  Relational Operator1/1 -> Data Type Conversion2/1
  1/relFreq2/1 -> Relational Operator1/2
  Product/1 -> Switch2/1, Switch1/3, Sum/1
  1/relFreq/1 -> Sum/2, Product/2
  1/relFreq1/1 -> Relational Operator/2

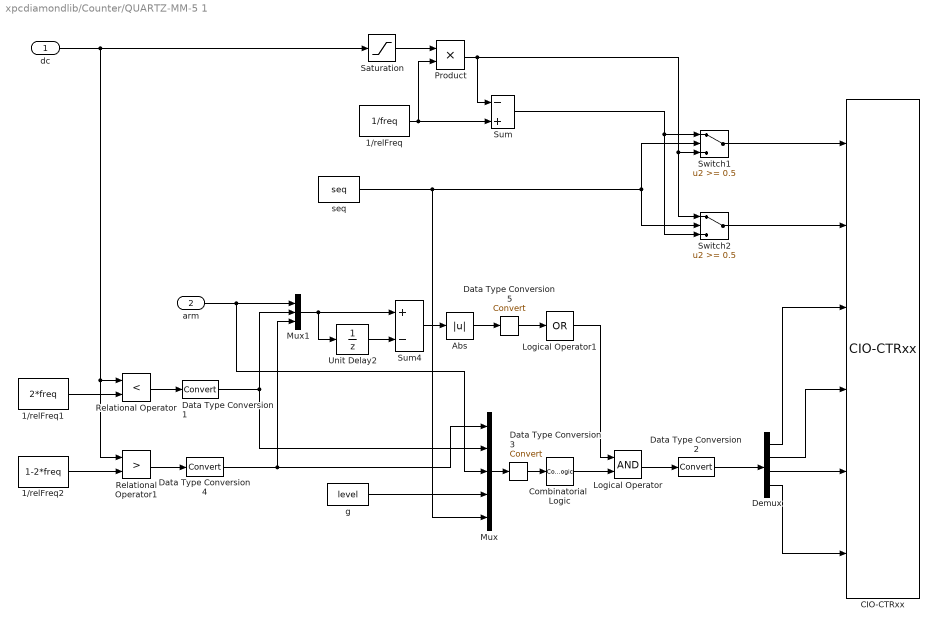
== system xpcdiamondlib/Counter/QUARTZ-MM-5 1 ==
  dc : Inport  LatchInput=off
  arm : Inport  Port=2  LatchInput=off
  1/relFreq : Constant  Value=1/freq
  1/relFreq1 : Constant  Value=2*freq
  1/relFreq2 : Constant  Value=1-2*freq
  Abs : Abs  SaturateOnIntegerOverflow=on
  "CIO-CTRxx " : xpcmeasurementcomputinglib/Counter/CIO-CTRxx   mastermode=MasterMode  countermode=CounterMode  init=Init  commands=Runtime  term=Term  ts=Ts  baseAddress=baseAddress
  Combinatorial  Logic : CombinatorialLogic  TruthTable=[0,0,1,0;0,0,1,0;0,0,0,1;0,0,0,1;0,1,0,0;1,0,0,0;0,1,0,0;1,0,0,0;0,0,1,0;0,0,1,0;0,0,0,1;0,0,0,1;0,0,1,0;0,0,1,0;0,0,1,0;0,0,1,0;0,0,1,0;0,0,1,0;0,0,0,1;0,0,0,1;0,0,0,1;0,0,0,1;0,0,0,1;0,0,0,1;0,0,0,0;0,0,0,0;0,0,0,0;0,0,0,0;0,0,0,0;0,0,0,0;0,0,0,0;0,0,0,0]
  Data Type Conversion1 : DataTypeConversion  OutDataTypeMode=double  SaturateOnIntegerOverflow=on  RndMeth=Zero
  Data Type Conversion2 : DataTypeConversion  SaturateOnIntegerOverflow=on  RndMeth=Zero
  Data Type Conversion3 : DataTypeConversion  SaturateOnIntegerOverflow=on  RndMeth=Zero
  Data Type Conversion4 : DataTypeConversion  OutDataTypeMode=double  SaturateOnIntegerOverflow=on  RndMeth=Zero
  Data Type Conversion5 : DataTypeConversion  SaturateOnIntegerOverflow=on  RndMeth=Zero
  Demux : Demux
  Logical Operator : Logic
  Logical Operator1 : Logic  Operator=OR  Inputs=1
  Mux : Mux  Inputs=5
  Mux1 : Mux  Inputs=3
  Product : Product  SaturateOnIntegerOverflow=on  InputSameDT=on
  Relational Operator : RelationalOperator  Operator=<  InputSameDT=on
  Relational Operator1 : RelationalOperator  Operator=>  InputSameDT=on
  Saturation : Saturate  UpperLimit=1-2*freq  LowerLimit=2*freq  ZeroCross=off
  Sum : Sum  Inputs=-+  SaturateOnIntegerOverflow=on  InputSameDT=on
  Sum4 : Sum  Inputs=+-  SaturateOnIntegerOverflow=on  InputSameDT=on
  Switch1 : Switch  Threshold=0.5  InputSameDT=on
  Switch2 : Switch  Threshold=0.5  InputSameDT=on
  Unit Delay2 : UnitDelay  X0=2  SampleTime=Ts
  g : Constant  Value=level
  seq : Constant  Value=seq
  wires:
  Data Type Conversion5/1 -> Logical Operator1/1
  Data Type Conversion3/1 -> Combinatorial  Logic/1
  Data Type Conversion2/1 -> Demux/1
  Data Type Conversion1/1 -> Mux1/2, Mux/2
  Data Type Conversion4/1 -> Mux1/3, Mux/1
  1/relFreq1/1 -> Relational Operator/2
  1/relFreq/1 -> Product/2, Sum/2
  Product/1 -> Sum/1, Switch1/3, Switch2/1
  1/relFreq2/1 -> Relational Operator1/2
  Relational Operator1/1 -> Data Type Conversion4/1
  Relational Operator/1 -> Data Type Conversion1/1
  Combinatorial  Logic/1 -> Logical Operator/2
  Logical Operator/1 -> Data Type Conversion2/1
  Unit Delay2/1 -> Sum4/2
  Sum4/1 -> Abs/1
  Logical Operator1/1 -> Logical Operator/1
  Demux/1 -> "CIO-CTRxx "/3
  Demux/2 -> "CIO-CTRxx "/4
  Demux/3 -> "CIO-CTRxx "/5
  Demux/4 -> "CIO-CTRxx "/6
  g/1 -> Mux/4
  seq/1 -> Switch1/2, Switch2/2, Mux/5
  Sum/1 -> Switch1/1, Switch2/3
  Saturation/1 -> Product/1
  dc/1 -> Saturation/1, Relational Operator/1, Relational Operator1/1
  Mux1/1 -> Sum4/1, Unit Delay2/1
  arm/1 -> Mux1/1, Mux/3
  Abs/1 -> Data Type Conversion5/1
  Mux/1 -> Data Type Conversion3/1
  Switch1/1 -> "CIO-CTRxx "/1
  Switch2/1 -> "CIO-CTRxx "/2

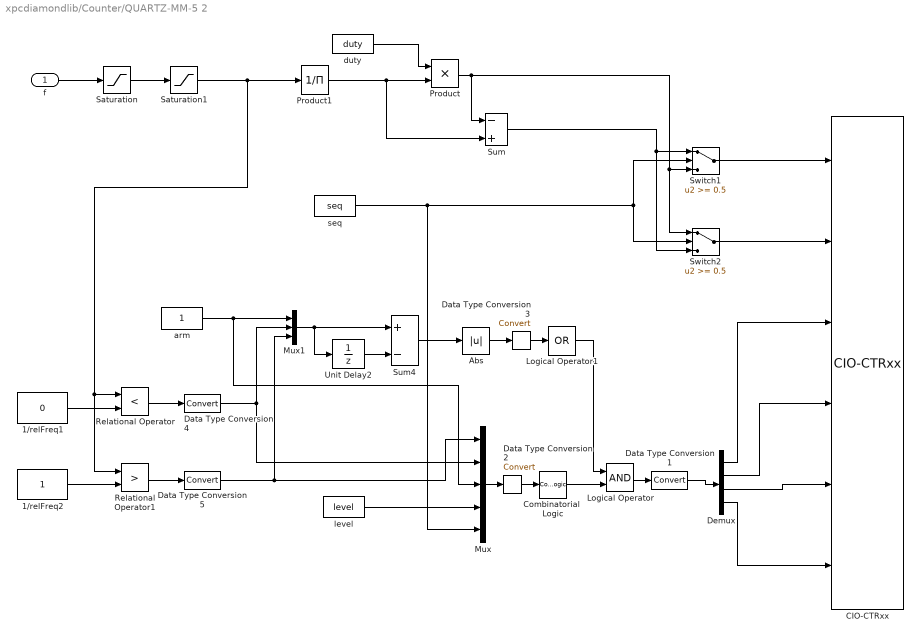
== system xpcdiamondlib/Counter/QUARTZ-MM-5 2 ==
  f : Inport  LatchInput=off
  1/relFreq1 : Constant  Value=0
  1/relFreq2 : Constant
  Abs : Abs  SaturateOnIntegerOverflow=on
  "CIO-CTRxx " : xpcmeasurementcomputinglib/Counter/CIO-CTRxx   mastermode=MasterMode  countermode=CounterMode  init=Init  commands=Runtime  term=Term  ts=Ts  baseAddress=baseAddress
  Combinatorial  Logic : CombinatorialLogic  TruthTable=[0,0,1,0;0,0,1,0;0,0,0,1;0,0,0,1;0,1,0,0;1,0,0,0;0,1,0,0;1,0,0,0;0,0,1,0;0,0,1,0;0,0,0,1;0,0,0,1;0,0,1,0;0,0,1,0;0,0,1,0;0,0,1,0;0,0,1,0;0,0,1,0;0,0,0,1;0,0,0,1;0,0,0,1;0,0,0,1;0,0,0,1;0,0,0,1;0,0,0,0;0,0,0,0;0,0,0,0;0,0,0,0;0,0,0,0;0,0,0,0;0,0,0,0;0,0,0,0]
  Data Type Conversion1 : DataTypeConversion  SaturateOnIntegerOverflow=on  RndMeth=Zero
  Data Type Conversion2 : DataTypeConversion  SaturateOnIntegerOverflow=on  RndMeth=Zero
  Data Type Conversion3 : DataTypeConversion  SaturateOnIntegerOverflow=on  RndMeth=Zero
  Data Type Conversion4 : DataTypeConversion  OutDataTypeMode=double  SaturateOnIntegerOverflow=on  RndMeth=Zero
  Data Type Conversion5 : DataTypeConversion  OutDataTypeMode=double  SaturateOnIntegerOverflow=on  RndMeth=Zero
  Demux : Demux
  Logical Operator : Logic
  Logical Operator1 : Logic  Operator=OR  Inputs=1
  Mux : Mux  Inputs=5
  Mux1 : Mux  Inputs=3
  Product : Product  SaturateOnIntegerOverflow=on  InputSameDT=on
  Product1 : Product  Inputs=/  SaturateOnIntegerOverflow=on  InputSameDT=on
  Relational Operator : RelationalOperator  Operator=<  InputSameDT=on
  Relational Operator1 : RelationalOperator  Operator=>  InputSameDT=on
  Saturation : Saturate  UpperLimit=duty/2  LowerLimit=duty/(2^16-1)  ZeroCross=off
  Saturation1 : Saturate  UpperLimit=(1-duty)/2  LowerLimit=(1-duty)/(2^16-1)  ZeroCross=off
  Sum : Sum  Inputs=-+  SaturateOnIntegerOverflow=on  InputSameDT=on
  Sum4 : Sum  Inputs=+-  SaturateOnIntegerOverflow=on  InputSameDT=on
  Switch1 : Switch  Threshold=0.5  InputSameDT=on
  Switch2 : Switch  Threshold=0.5  InputSameDT=on
  Unit Delay2 : UnitDelay  X0=2  SampleTime=Ts
  arm : Constant
  duty : Constant  Value=duty
  level : Constant  Value=level
  seq : Constant  Value=seq
  wires:
  Data Type Conversion5/1 -> Mux1/3, Mux/1
  Data Type Conversion4/1 -> Mux1/2, Mux/2
  Data Type Conversion3/1 -> Logical Operator1/1
  Data Type Conversion2/1 -> Combinatorial  Logic/1
  Data Type Conversion1/1 -> Demux/1
  1/relFreq1/1 -> Relational Operator/2
  Product/1 -> Sum/1, Switch1/3, Switch2/1
  1/relFreq2/1 -> Relational Operator1/2
  Relational Operator1/1 -> Data Type Conversion5/1
  Relational Operator/1 -> Data Type Conversion4/1
  Combinatorial  Logic/1 -> Logical Operator/2
  Logical Operator/1 -> Data Type Conversion1/1
  Unit Delay2/1 -> Sum4/2
  Sum4/1 -> Abs/1
  Logical Operator1/1 -> Logical Operator/1
  Demux/1 -> "CIO-CTRxx "/3
  Demux/2 -> "CIO-CTRxx "/4
  Demux/3 -> "CIO-CTRxx "/5
  Demux/4 -> "CIO-CTRxx "/6
  level/1 -> Mux/4
  Switch1/1 -> "CIO-CTRxx "/1
  Switch2/1 -> "CIO-CTRxx "/2
  seq/1 -> Switch1/2, Switch2/2, Mux/5
  Sum/1 -> Switch1/1, Switch2/3
  Saturation/1 -> Saturation1/1
  f/1 -> Saturation/1
  Mux1/1 -> Sum4/1, Unit Delay2/1
  arm/1 -> Mux1/1, Mux/3
  Abs/1 -> Data Type Conversion3/1
  Mux/1 -> Data Type Conversion2/1
  Saturation1/1 -> Product1/1, Relational Operator1/1, Relational Operator/1
  duty/1 -> Product/1
  Product1/1 -> Product/2, Sum/2

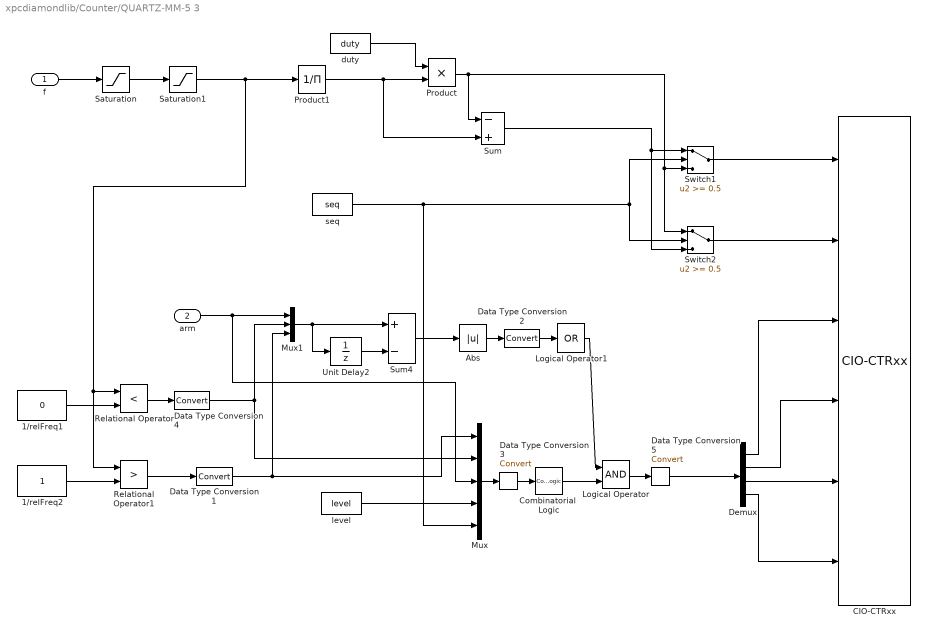
== system xpcdiamondlib/Counter/QUARTZ-MM-5 3 ==
  f : Inport  LatchInput=off
  arm : Inport  Port=2  LatchInput=off
  1/relFreq1 : Constant  Value=0
  1/relFreq2 : Constant
  Abs : Abs  SaturateOnIntegerOverflow=on
  "CIO-CTRxx " : xpcmeasurementcomputinglib/Counter/CIO-CTRxx   mastermode=MasterMode  countermode=CounterMode  init=Init  commands=Runtime  term=Term  ts=Ts  baseAddress=baseAddress
  Combinatorial  Logic : CombinatorialLogic  TruthTable=[0,0,1,0;0,0,1,0;0,0,0,1;0,0,0,1;0,1,0,0;1,0,0,0;0,1,0,0;1,0,0,0;0,0,1,0;0,0,1,0;0,0,0,1;0,0,0,1;0,0,1,0;0,0,1,0;0,0,1,0;0,0,1,0;0,0,1,0;0,0,1,0;0,0,0,1;0,0,0,1;0,0,0,1;0,0,0,1;0,0,0,1;0,0,0,1;0,0,0,0;0,0,0,0;0,0,0,0;0,0,0,0;0,0,0,0;0,0,0,0;0,0,0,0;0,0,0,0]
  Data Type Conversion1 : DataTypeConversion  OutDataTypeMode=double  SaturateOnIntegerOverflow=on  RndMeth=Zero
  Data Type Conversion2 : DataTypeConversion  SaturateOnIntegerOverflow=on  RndMeth=Zero
  Data Type Conversion3 : DataTypeConversion  SaturateOnIntegerOverflow=on  RndMeth=Zero
  Data Type Conversion4 : DataTypeConversion  OutDataTypeMode=double  SaturateOnIntegerOverflow=on  RndMeth=Zero
  Data Type Conversion5 : DataTypeConversion  SaturateOnIntegerOverflow=on  RndMeth=Zero
  Demux : Demux
  Logical Operator : Logic
  Logical Operator1 : Logic  Operator=OR  Inputs=1
  Mux : Mux  Inputs=5
  Mux1 : Mux  Inputs=3
  Product : Product  SaturateOnIntegerOverflow=on  InputSameDT=on
  Product1 : Product  Inputs=/  SaturateOnIntegerOverflow=on  InputSameDT=on
  Relational Operator : RelationalOperator  Operator=<  InputSameDT=on
  Relational Operator1 : RelationalOperator  Operator=>  InputSameDT=on
  Saturation : Saturate  UpperLimit=duty/2  LowerLimit=duty/(2^16-1)  ZeroCross=off
  Saturation1 : Saturate  UpperLimit=(1-duty)/2  LowerLimit=(1-duty)/(2^16-1)  ZeroCross=off
  Sum : Sum  Inputs=-+  SaturateOnIntegerOverflow=on  InputSameDT=on
  Sum4 : Sum  Inputs=+-  SaturateOnIntegerOverflow=on  InputSameDT=on
  Switch1 : Switch  Threshold=0.5  InputSameDT=on
  Switch2 : Switch  Threshold=0.5  InputSameDT=on
  Unit Delay2 : UnitDelay  X0=2  SampleTime=Ts
  duty : Constant  Value=duty
  level : Constant  Value=level
  seq : Constant  Value=seq
  wires:
  Data Type Conversion5/1 -> Demux/1
  Data Type Conversion3/1 -> Combinatorial  Logic/1
  Data Type Conversion2/1 -> Logical Operator1/1
  Data Type Conversion1/1 -> Mux1/3, Mux/1
  Data Type Conversion4/1 -> Mux1/2, Mux/2
  1/relFreq1/1 -> Relational Operator/2
  Product/1 -> Sum/1, Switch1/3, Switch2/1
  1/relFreq2/1 -> Relational Operator1/2
  Relational Operator1/1 -> Data Type Conversion1/1
  Relational Operator/1 -> Data Type Conversion4/1
  Combinatorial  Logic/1 -> Logical Operator/2
  Logical Operator/1 -> Data Type Conversion5/1
  Unit Delay2/1 -> Sum4/2
  Sum4/1 -> Abs/1
  Logical Operator1/1 -> Logical Operator/1
  Demux/1 -> "CIO-CTRxx "/3
  Demux/2 -> "CIO-CTRxx "/4
  Demux/3 -> "CIO-CTRxx "/5
  Demux/4 -> "CIO-CTRxx "/6
  level/1 -> Mux/4
  Switch1/1 -> "CIO-CTRxx "/1
  Switch2/1 -> "CIO-CTRxx "/2
  seq/1 -> Switch1/2, Switch2/2, Mux/5
  Sum/1 -> Switch1/1, Switch2/3
  Saturation/1 -> Saturation1/1
  f/1 -> Saturation/1
  Mux1/1 -> Sum4/1, Unit Delay2/1
  arm/1 -> Mux1/1, Mux/3
  Abs/1 -> Data Type Conversion2/1
  Mux/1 -> Data Type Conversion3/1
  Saturation1/1 -> Product1/1, Relational Operator1/1, Relational Operator/1
  duty/1 -> Product/1
  Product1/1 -> Product/2, Sum/2

== system xpcdiamondlib/Counter/QUARTZ-MM-5 4 ==
  "CIO-CTRxx " : xpcmeasurementcomputinglib/Counter/CIO-CTRxx   mastermode=MasterMode  countermode=CounterMode  init=Init  commands=Runtime  term=Term  ts=Ts  baseAddress=baseAddress
  Demux : Demux  Outputs=2
  Product : Product  Inputs=/  SaturateOnIntegerOverflow=on  InputSameDT=on
  Product1 : Product  Inputs=**  SaturateOnIntegerOverflow=on  InputSameDT=on
  f : Outport
  dc : Outport  Port=2
  wires:
  Product1/1 -> dc/1
  Product/1 -> Product1/2, f/1
  Demux/2 -> Product/1
  Demux/1 -> Product1/1
  "CIO-CTRxx "/1 -> Demux/1

== system xpcdiamondlib/Counter/QUARTZ-MM-5 5 ==
  "CIO-CTRxx " : xpcmeasurementcomputinglib/Counter/CIO-CTRxx   mastermode=MasterMode  countermode=CounterMode  init=Init  commands=Runtime  term=Term  ts=Ts  baseAddress=baseAddress
  Product : Product  Inputs=/  SaturateOnIntegerOverflow=on  InputSameDT=on
  f : Outport
  wires:
  Product/1 -> f/1
  "CIO-CTRxx "/1 -> Product/1
